simulink model "speed_error_unit_test"  (R2024a)
settings: Solver=VariableStepAuto  StartTime=0.0  StopTime=10.0  RelTol=1e-3
settings Model: Creator=lucap  LastModifiedBy=lucap

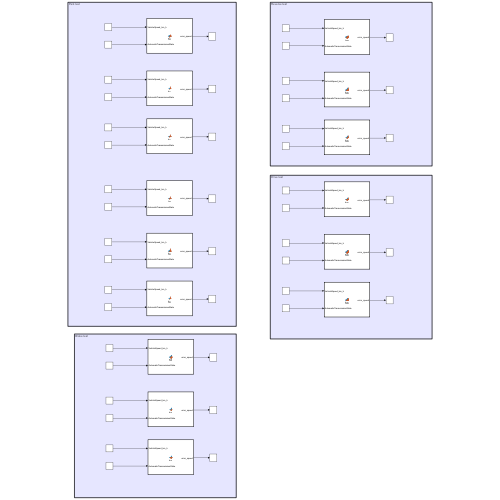
[thumbnail: Simulink's stored preview of the top-level diagram]
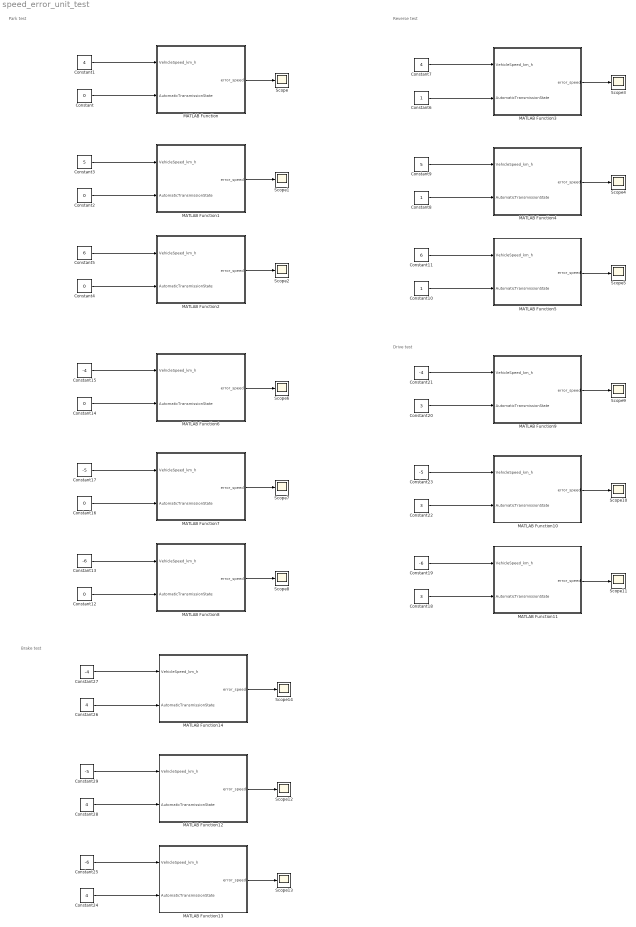
== system speed_error_unit_test ==
  note: Park test
  note: Reverse test
  note: Drive test
  note: Brake test
  Constant{,2,4,12,14,16} (6 alike) : Constant  Value=0  OutDataTypeStr=int32
  Constant1 : Constant  Value=4
  Constant10 : Constant  OutDataTypeStr=int32
  Constant11 : Constant  Value=6
  Constant13 : Constant  Value=-6
  Constant15 : Constant  Value=-4
  Constant17 : Constant  Value=-5
  Constant18 : Constant  Value=3  OutDataTypeStr=int32
  Constant19 : Constant  Value=-6
  Constant20 : Constant  Value=3  OutDataTypeStr=int32
  Constant21 : Constant  Value=-4
  Constant22 : Constant  Value=3  OutDataTypeStr=int32
  Constant23 : Constant  Value=-5
  Constant24 : Constant  Value=4  OutDataTypeStr=int32
  Constant25 : Constant  Value=-6
  Constant26 : Constant  Value=4  OutDataTypeStr=int32
  Constant27 : Constant  Value=-4
  Constant28 : Constant  Value=4  OutDataTypeStr=int32
  Constant29 : Constant  Value=-5
  Constant3 : Constant  Value=5
  Constant5 : Constant  Value=6
  Constant6 : Constant  OutDataTypeStr=int32
  Constant7 : Constant  Value=4
  Constant8 : Constant  OutDataTypeStr=int32
  Constant9 : Constant  Value=5
  MATLAB Function : MATLAB Function  TreatAsAtomicUnit=on
  MATLAB Function1 : MATLAB Function  TreatAsAtomicUnit=on
  MATLAB Function10 : MATLAB Function  TreatAsAtomicUnit=on
  MATLAB Function11 : MATLAB Function  TreatAsAtomicUnit=on
  MATLAB Function12 : MATLAB Function  TreatAsAtomicUnit=on
  MATLAB Function13 : MATLAB Function  TreatAsAtomicUnit=on
  MATLAB Function14 : MATLAB Function  TreatAsAtomicUnit=on
  MATLAB Function2 : MATLAB Function  TreatAsAtomicUnit=on
  MATLAB Function3 : MATLAB Function  TreatAsAtomicUnit=on
  MATLAB Function4 : MATLAB Function  TreatAsAtomicUnit=on
  MATLAB Function5 : MATLAB Function  TreatAsAtomicUnit=on
  MATLAB Function6 : MATLAB Function  TreatAsAtomicUnit=on
  MATLAB Function7 : MATLAB Function  TreatAsAtomicUnit=on
  MATLAB Function8 : MATLAB Function  TreatAsAtomicUnit=on
  MATLAB Function9 : MATLAB Function  TreatAsAtomicUnit=on
  Scope{,1..14} (15 alike) : Scope
  wires:
  Constant1/1 -> MATLAB Function/1(VehicleSpeed_km_h)
  Constant/1 -> MATLAB Function/2(AutomaticTransmissionState)
  MATLAB Function/1(error_speed) -> Scope/1
  Constant3/1 -> MATLAB Function1/1(VehicleSpeed_km_h)
  MATLAB Function1/1(error_speed) -> Scope1/1
  Constant5/1 -> MATLAB Function2/1(VehicleSpeed_km_h)
  MATLAB Function2/1(error_speed) -> Scope2/1
  Constant2/1 -> MATLAB Function1/2(AutomaticTransmissionState)
  Constant4/1 -> MATLAB Function2/2(AutomaticTransmissionState)
  Constant10/1 -> MATLAB Function5/2(AutomaticTransmissionState)
  Constant9/1 -> MATLAB Function4/1(VehicleSpeed_km_h)
  Constant6/1 -> MATLAB Function3/2(AutomaticTransmissionState)
  Constant8/1 -> MATLAB Function4/2(AutomaticTransmissionState)
  MATLAB Function3/1(error_speed) -> Scope3/1
  Constant7/1 -> MATLAB Function3/1(VehicleSpeed_km_h)
  MATLAB Function5/1(error_speed) -> Scope5/1
  Constant11/1 -> MATLAB Function5/1(VehicleSpeed_km_h)
  MATLAB Function4/1(error_speed) -> Scope4/1
  Constant13/1 -> MATLAB Function8/1(VehicleSpeed_km_h)
  MATLAB Function7/1(error_speed) -> Scope7/1
  Constant15/1 -> MATLAB Function6/1(VehicleSpeed_km_h)
  MATLAB Function8/1(error_speed) -> Scope8/1
  Constant14/1 -> MATLAB Function6/2(AutomaticTransmissionState)
  MATLAB Function6/1(error_speed) -> Scope6/1
  Constant16/1 -> MATLAB Function7/2(AutomaticTransmissionState)
  Constant17/1 -> MATLAB Function7/1(VehicleSpeed_km_h)
  Constant12/1 -> MATLAB Function8/2(AutomaticTransmissionState)
  MATLAB Function10/1(error_speed) -> Scope10/1
  Constant22/1 -> MATLAB Function10/2(AutomaticTransmissionState)
  Constant20/1 -> MATLAB Function9/2(AutomaticTransmissionState)
  MATLAB Function11/1(error_speed) -> Scope11/1
  Constant21/1 -> MATLAB Function9/1(VehicleSpeed_km_h)
  Constant19/1 -> MATLAB Function11/1(VehicleSpeed_km_h)
  Constant18/1 -> MATLAB Function11/2(AutomaticTransmissionState)
  MATLAB Function9/1(error_speed) -> Scope9/1
  Constant23/1 -> MATLAB Function10/1(VehicleSpeed_km_h)
  MATLAB Function13/1(error_speed) -> Scope13/1
  MATLAB Function14/1(error_speed) -> Scope14/1
  Constant24/1 -> MATLAB Function13/2(AutomaticTransmissionState)
  Constant28/1 -> MATLAB Function12/2(AutomaticTransmissionState)
  Constant27/1 -> MATLAB Function14/1(VehicleSpeed_km_h)
  Constant26/1 -> MATLAB Function14/2(AutomaticTransmissionState)
  MATLAB Function12/1(error_speed) -> Scope12/1
  Constant29/1 -> MATLAB Function12/1(VehicleSpeed_km_h)
  Constant25/1 -> MATLAB Function13/1(VehicleSpeed_km_h)

== matlab function speed_error_unit_test/MATLAB Function12 ==
  data: VehicleSpeed_km_h input; AutomaticTransmissionState input; error_speed output
function error_speed = fcn(VehicleSpeed_km_h, AutomaticTransmissionState)

if AutomaticTransmissionState == TransmissionState.Reverse && VehicleSpeed_km_h >= 5
        error_speed = boolean(1);
elseif AutomaticTransmissionState == TransmissionState.Park && abs(VehicleSpeed_km_h) >= 5
        error_speed = boolean(1);
elseif AutomaticTransmissionState == TransmissionState.Drive && VehicleSpeed_km_h <= -5
        error_speed = boolean(1);
elseif AutomaticTransmissionState == TransmissionState.Brake && VehicleSpeed_km_h <= -5
        error_speed = boolean(1);
else
    error_speed = boolean(0);
end

== matlab function speed_error_unit_test/MATLAB Function13 ==
  data: VehicleSpeed_km_h input; AutomaticTransmissionState input; error_speed output
function error_speed = fcn(VehicleSpeed_km_h, AutomaticTransmissionState)

if AutomaticTransmissionState == TransmissionState.Reverse && VehicleSpeed_km_h >= 5
        error_speed = boolean(1);
elseif AutomaticTransmissionState == TransmissionState.Park && abs(VehicleSpeed_km_h) >= 5
        error_speed = boolean(1);
elseif AutomaticTransmissionState == TransmissionState.Drive && VehicleSpeed_km_h <= -5
        error_speed = boolean(1);
elseif AutomaticTransmissionState == TransmissionState.Brake && VehicleSpeed_km_h <= -5
        error_speed = boolean(1);
else
    error_speed = boolean(0);
end

== matlab function speed_error_unit_test/MATLAB Function14 ==
  data: VehicleSpeed_km_h input; AutomaticTransmissionState input; error_speed output
function error_speed = fcn(VehicleSpeed_km_h, AutomaticTransmissionState)

if AutomaticTransmissionState == TransmissionState.Reverse && VehicleSpeed_km_h >= 5
        error_speed = boolean(1);
elseif AutomaticTransmissionState == TransmissionState.Park && abs(VehicleSpeed_km_h) >= 5
        error_speed = boolean(1);
elseif AutomaticTransmissionState == TransmissionState.Drive && VehicleSpeed_km_h <= -5
        error_speed = boolean(1);
elseif AutomaticTransmissionState == TransmissionState.Brake && VehicleSpeed_km_h <= -5
        error_speed = boolean(1);
else
    error_speed = boolean(0);
end

== matlab function speed_error_unit_test/MATLAB Function1 ==
  data: VehicleSpeed_km_h input; AutomaticTransmissionState input; error_speed output
function error_speed = fcn(VehicleSpeed_km_h, AutomaticTransmissionState)

if AutomaticTransmissionState == TransmissionState.Reverse && VehicleSpeed_km_h >= 5
        error_speed = boolean(1);
elseif AutomaticTransmissionState == TransmissionState.Park && abs(VehicleSpeed_km_h) >= 5
        error_speed = boolean(1);
elseif AutomaticTransmissionState == TransmissionState.Drive && VehicleSpeed_km_h <= -5
        error_speed = boolean(1);
elseif AutomaticTransmissionState == TransmissionState.Brake && VehicleSpeed_km_h <= -5
        error_speed = boolean(1);
else
    error_speed = boolean(0);
end

== matlab function speed_error_unit_test/MATLAB Function2 ==
  data: VehicleSpeed_km_h input; AutomaticTransmissionState input; error_speed output
function error_speed = fcn(VehicleSpeed_km_h, AutomaticTransmissionState)

if AutomaticTransmissionState == TransmissionState.Reverse && VehicleSpeed_km_h >= 5
        error_speed = boolean(1);
elseif AutomaticTransmissionState == TransmissionState.Park && abs(VehicleSpeed_km_h) >= 5
        error_speed = boolean(1);
elseif AutomaticTransmissionState == TransmissionState.Drive && VehicleSpeed_km_h <= -5
        error_speed = boolean(1);
elseif AutomaticTransmissionState == TransmissionState.Brake && VehicleSpeed_km_h <= -5
        error_speed = boolean(1);
else
    error_speed = boolean(0);
end

== matlab function speed_error_unit_test/MATLAB Function3 ==
  data: VehicleSpeed_km_h input; AutomaticTransmissionState input; error_speed output
function error_speed = fcn(VehicleSpeed_km_h, AutomaticTransmissionState)

if AutomaticTransmissionState == TransmissionState.Reverse && VehicleSpeed_km_h >= 5
        error_speed = boolean(1);
elseif AutomaticTransmissionState == TransmissionState.Park && abs(VehicleSpeed_km_h) >= 5
        error_speed = boolean(1);
elseif AutomaticTransmissionState == TransmissionState.Drive && VehicleSpeed_km_h <= -5
        error_speed = boolean(1);
elseif AutomaticTransmissionState == TransmissionState.Brake && VehicleSpeed_km_h <= -5
        error_speed = boolean(1);
else
    error_speed = boolean(0);
end

== matlab function speed_error_unit_test/MATLAB Function4 ==
  data: VehicleSpeed_km_h input; AutomaticTransmissionState input; error_speed output
function error_speed = fcn(VehicleSpeed_km_h, AutomaticTransmissionState)

if AutomaticTransmissionState == TransmissionState.Reverse && VehicleSpeed_km_h >= 5
        error_speed = boolean(1);
elseif AutomaticTransmissionState == TransmissionState.Park && abs(VehicleSpeed_km_h) >= 5
        error_speed = boolean(1);
elseif AutomaticTransmissionState == TransmissionState.Drive && VehicleSpeed_km_h <= -5
        error_speed = boolean(1);
elseif AutomaticTransmissionState == TransmissionState.Brake && VehicleSpeed_km_h <= -5
        error_speed = boolean(1);
else
    error_speed = boolean(0);
end

== matlab function speed_error_unit_test/MATLAB Function5 ==
  data: VehicleSpeed_km_h input; AutomaticTransmissionState input; error_speed output
function error_speed = fcn(VehicleSpeed_km_h, AutomaticTransmissionState)

if AutomaticTransmissionState == TransmissionState.Reverse && VehicleSpeed_km_h >= 5
        error_speed = boolean(1);
elseif AutomaticTransmissionState == TransmissionState.Park && abs(VehicleSpeed_km_h) >= 5
        error_speed = boolean(1);
elseif AutomaticTransmissionState == TransmissionState.Drive && VehicleSpeed_km_h <= -5
        error_speed = boolean(1);
elseif AutomaticTransmissionState == TransmissionState.Brake && VehicleSpeed_km_h <= -5
        error_speed = boolean(1);
else
    error_speed = boolean(0);
end

== matlab function speed_error_unit_test/MATLAB Function6 ==
  data: VehicleSpeed_km_h input; AutomaticTransmissionState input; error_speed output
function error_speed = fcn(VehicleSpeed_km_h, AutomaticTransmissionState)

if AutomaticTransmissionState == TransmissionState.Reverse && VehicleSpeed_km_h >= 5
        error_speed = boolean(1);
elseif AutomaticTransmissionState == TransmissionState.Park && abs(VehicleSpeed_km_h) >= 5
        error_speed = boolean(1);
elseif AutomaticTransmissionState == TransmissionState.Drive && VehicleSpeed_km_h <= -5
        error_speed = boolean(1);
elseif AutomaticTransmissionState == TransmissionState.Brake && VehicleSpeed_km_h <= -5
        error_speed = boolean(1);
else
    error_speed = boolean(0);
end

== matlab function speed_error_unit_test/MATLAB Function7 ==
  data: VehicleSpeed_km_h input; AutomaticTransmissionState input; error_speed output
function error_speed = fcn(VehicleSpeed_km_h, AutomaticTransmissionState)

if AutomaticTransmissionState == TransmissionState.Reverse && VehicleSpeed_km_h >= 5
        error_speed = boolean(1);
elseif AutomaticTransmissionState == TransmissionState.Park && abs(VehicleSpeed_km_h) >= 5
        error_speed = boolean(1);
elseif AutomaticTransmissionState == TransmissionState.Drive && VehicleSpeed_km_h <= -5
        error_speed = boolean(1);
elseif AutomaticTransmissionState == TransmissionState.Brake && VehicleSpeed_km_h <= -5
        error_speed = boolean(1);
else
    error_speed = boolean(0);
end

== matlab function speed_error_unit_test/MATLAB Function8 ==
  data: VehicleSpeed_km_h input; AutomaticTransmissionState input; error_speed output
function error_speed = fcn(VehicleSpeed_km_h, AutomaticTransmissionState)

if AutomaticTransmissionState == TransmissionState.Reverse && VehicleSpeed_km_h >= 5
        error_speed = boolean(1);
elseif AutomaticTransmissionState == TransmissionState.Park && abs(VehicleSpeed_km_h) >= 5
        error_speed = boolean(1);
elseif AutomaticTransmissionState == TransmissionState.Drive && VehicleSpeed_km_h <= -5
        error_speed = boolean(1);
elseif AutomaticTransmissionState == TransmissionState.Brake && VehicleSpeed_km_h <= -5
        error_speed = boolean(1);
else
    error_speed = boolean(0);
end

== matlab function speed_error_unit_test/MATLAB Function ==
  data: VehicleSpeed_km_h input; AutomaticTransmissionState input; error_speed output
function error_speed = fcn(VehicleSpeed_km_h, AutomaticTransmissionState)

if AutomaticTransmissionState == TransmissionState.Reverse && VehicleSpeed_km_h >= 5
        error_speed = boolean(1);
elseif AutomaticTransmissionState == TransmissionState.Park && abs(VehicleSpeed_km_h) >= 5
        error_speed = boolean(1);
elseif AutomaticTransmissionState == TransmissionState.Drive && VehicleSpeed_km_h <= -5
        error_speed = boolean(1);
elseif AutomaticTransmissionState == TransmissionState.Brake && VehicleSpeed_km_h <= -5
        error_speed = boolean(1);
else
    error_speed = boolean(0);
end

== matlab function speed_error_unit_test/MATLAB Function10 ==
  data: VehicleSpeed_km_h input; AutomaticTransmissionState input; error_speed output
function error_speed = fcn(VehicleSpeed_km_h, AutomaticTransmissionState)

if AutomaticTransmissionState == TransmissionState.Reverse && VehicleSpeed_km_h >= 5
        error_speed = boolean(1);
elseif AutomaticTransmissionState == TransmissionState.Park && abs(VehicleSpeed_km_h) >= 5
        error_speed = boolean(1);
elseif AutomaticTransmissionState == TransmissionState.Drive && VehicleSpeed_km_h <= -5
        error_speed = boolean(1);
elseif AutomaticTransmissionState == TransmissionState.Brake && VehicleSpeed_km_h <= -5
        error_speed = boolean(1);
else
    error_speed = boolean(0);
end

== matlab function speed_error_unit_test/MATLAB Function11 ==
  data: VehicleSpeed_km_h input; AutomaticTransmissionState input; error_speed output
function error_speed = fcn(VehicleSpeed_km_h, AutomaticTransmissionState)

if AutomaticTransmissionState == TransmissionState.Reverse && VehicleSpeed_km_h >= 5
        error_speed = boolean(1);
elseif AutomaticTransmissionState == TransmissionState.Park && abs(VehicleSpeed_km_h) >= 5
        error_speed = boolean(1);
elseif AutomaticTransmissionState == TransmissionState.Drive && VehicleSpeed_km_h <= -5
        error_speed = boolean(1);
elseif AutomaticTransmissionState == TransmissionState.Brake && VehicleSpeed_km_h <= -5
        error_speed = boolean(1);
else
    error_speed = boolean(0);
end

== matlab function speed_error_unit_test/MATLAB Function9 ==
  data: VehicleSpeed_km_h input; AutomaticTransmissionState input; error_speed output
function error_speed = fcn(VehicleSpeed_km_h, AutomaticTransmissionState)

if AutomaticTransmissionState == TransmissionState.Reverse && VehicleSpeed_km_h >= 5
        error_speed = boolean(1);
elseif AutomaticTransmissionState == TransmissionState.Park && abs(VehicleSpeed_km_h) >= 5
        error_speed = boolean(1);
elseif AutomaticTransmissionState == TransmissionState.Drive && VehicleSpeed_km_h <= -5
        error_speed = boolean(1);
elseif AutomaticTransmissionState == TransmissionState.Brake && VehicleSpeed_km_h <= -5
        error_speed = boolean(1);
else
    error_speed = boolean(0);
end
